simulink model "Spectrum_Analizer"  (R2022a)
settings: Solver=VariableStepAuto  StartTime=0.0  StopTime=100  RelTol=1e-3
InitFcn:
  | ts3=0.001;
  | dt=0.001;
libraries: dspsrcs4 x1, simulink x1
settings Model: Creator=TC16766  LastModifiedBy=ohadformanair
settings SolverCC: AlgebraicLoopSolver=TrustRegion
settings DebuggingCC: UnconnectedInputMsg=warning  UnconnectedOutputMsg=warning  UnconnectedLineMsg=warning  SFMachineParentedDataDiag=warning
settings RTWCC: DLArmComputeVersion=19.05

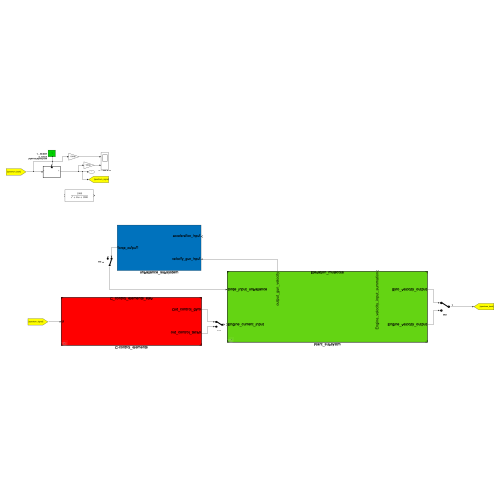
[thumbnail: Simulink's stored preview of the top-level diagram]
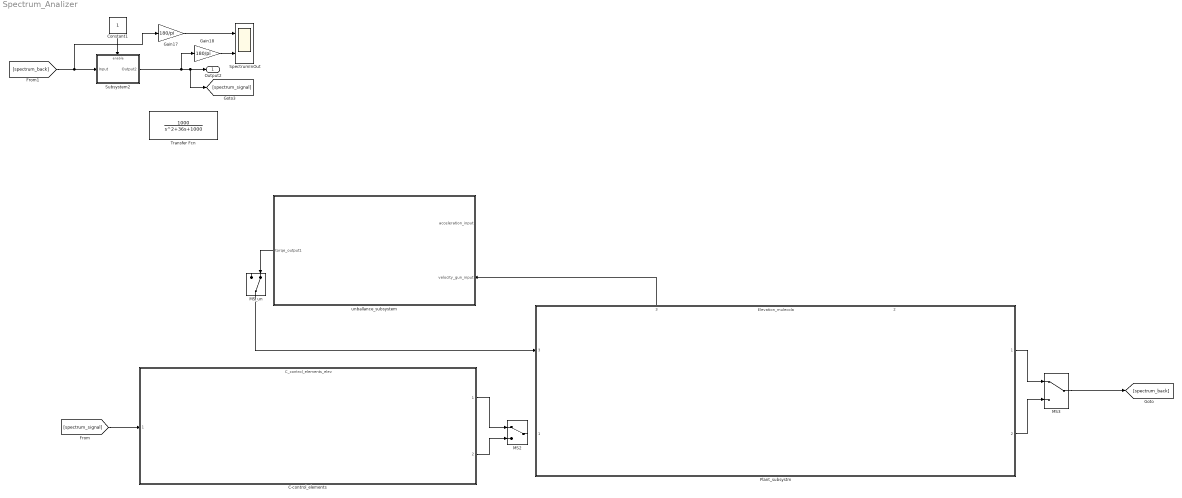
== system Spectrum_Analizer ==
  C-control_elements : ModelReference  ModelNameDialog=C_control_elements_elev  SimulationMode=Normal  ModelReferenceVersion=1.111
  Constant1 : Constant  OutDataTypeStr=boolean
      settings: AttributesFormatString=1 - START\n0 -STOP\ninternal spectrum
      settings: OpenFcn=|
      | if get_param(gcbh,'value')-48 set_param(gcbh,'value','0','backgroundcolor','red');
      | else set_param(gcbh,'value','1','backgroundcolor','green');
      | end
  Gain17 : Gain  Gain=180/pi
  Gain18 : Gain  Gain=180/pi
  MS2 : ManualSwitch
  MS3 : ManualSwitch
  MS_un : ManualSwitch  CurrentSetting=0
  Plant_subsystm : ModelReference  ModelNameDialog=Elevation_mulecola.slx  SimulationMode=Normal  ModelReferenceVersion=1.74
      settings: PortSchema="{\"entries\":[{\"content\":{\"sides\":[{\"content\":{\"connectorIds\":[\"In3\",\"In1\"]},\"type\":\"ConnectorPlacement.EquallySpacedRectSide\",\"uuid\":\"5c3be150-06c1-4b04-81d4-c89054a50b58\"},{\"content\":{\"connectorIds\":[\"Out1\",\"Out2\"],\"side\":\"RIGHT\"},\"type\":\"ConnectorPlacement.EquallySpacedRectSide\",\"uuid\":\"5dfcaa34-ef70-477d-9189-6856ebc4bbcf\"},{\"content\":{\"connectorIds\":[\"Out3\",\"In2\"],\"side\":\"TOP\"},\"type\":\"ConnectorPlacement.EquallySpacedRectSide\",\"uuid\":\"06d3d264-a507-4be0-8bff-1d5586be5fcb\"}]},\"type\":\"ConnectorPlacement.EquallySpacedConnector\",\"uuid\":\"1f4e30e1-d134-49fc-8bd6-0842cd83f06c\"}],\"packageUris\":[\"http://schema.mathworks.com/mf0/Connector/R2020b\"],\"version\":\"1.0\"}"
  SpectrumInOut : Scope  NumInputPorts=2
  Subsystem2 : Subsystem  mask{GAIN=1%2*pi/180%0.5*pi/180, InitFreq=1, TargetTime=100, FreqAtTime=100}
      mask prompts: InitFreq "INITIAL FREQUENCY"; TargetTime "Target Time"; FreqAtTime "Frequency at Time"
  Transfer Fcn : TransferFcn  Numerator=[1000]  Denominator=[1 36 1000]
  unballance_subsystem : Subsystem
      settings: PortSchema="{\"entries\":[{\"content\":{\"sides\":[{\"content\":{\"connectorIds\":[\"Out1\"]},\"type\":\"ConnectorPlacement.EquallySpacedRectSide\",\"uuid\":\"c3cd5407-f455-47fb-bed5-acab7b307edd\"},{\"content\":{\"connectorIds\":[\"In1\",\"In2\"],\"side\":\"RIGHT\"},\"type\":\"ConnectorPlacement.EquallySpacedRectSide\",\"uuid\":\"6fee87de-46ca-4c43-9525-17ad0f41a606\"},{\"content\":{\"connectorIds\":[],\"side\":\"TOP\"},\"type\":\"ConnectorPlacement.EquallySpacedRectSide\",\"uuid\":\"ba4483d7-ae58-474a-ba17-43cd832aaa5a\"},{\"content\":{\"connectorIds\":[],\"side\":\"BOTTOM\"},\"type\":\"ConnectorPlacement.EquallySpacedRectSide\",\"uuid\":\"48dc55aa-c39e-4e9a-95dc-6c3e56dde9f8\"}]},\"type\":\"ConnectorPlacement.EquallySpacedConnector\",\"uuid\":\"1afecaf5-de5a-4863-97c1-6af15bef8986\"}],\"packageUris\":[\"http://schema.mathworks.com/mf0/Connector/R2020b\"],\"version\":\"1.0\"}"
  Output2 : Outport
  wires:
  Subsystem2/1(Output2) -> [spectrum_signal], Output2/1, Gain18/1
  Gain17/1 -> SpectrumInOut/1
  Gain18/1 -> SpectrumInOut/2
  [spectrum_back] -> Gain17/1, Subsystem2/1(Input)
  Constant1/1 -> Subsystem2/Enable
  C-control_elements/2 -> MS2/2
  unballance_subsystem/1(torqe_output1) -> MS_un/2
  C-control_elements/1 -> MS2/1
  Plant_subsystm/3 -> unballance_subsystem/2(velocity_gun_input)
  MS_un/1 -> Plant_subsystm/3
  Plant_subsystm/1 -> MS3/1
  Plant_subsystm/2 -> MS3/2
  [spectrum_signal] -> C-control_elements/1
  MS3/1 -> [spectrum_back]

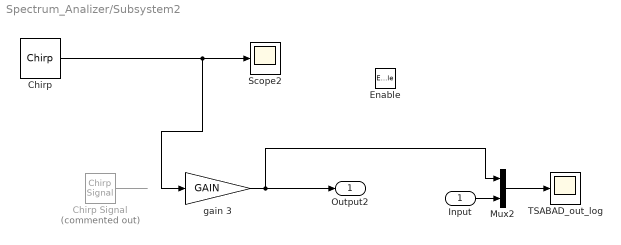
== system Spectrum_Analizer/Subsystem2 ==
  Input : Inport
  Enable : EnablePort  StatesWhenEnabling=reset
  Chirp : dspsrcs4/Chirp  sweep=Quadratic  mode=Unidirectional  f0=1  f1=FreqAtTime  t1=TargetTime  Tsweep=TargetTime  phase=0  Ts=1/100000  spf=1  datatype=Double  OutputFrames=off
  Chirp Signal : simulink/Sources/Chirp Signal  Commented=on  f1=InitFreq  T=TargetTime  f2=FreqAtTime
  Mux2 : Mux  Inputs=2
  Scope2 : Scope
  TSABAD_out_log : Scope
  gain 3 : Gain  Gain=GAIN  SaturateOnIntegerOverflow=on  SampleTime=ts3  OutDataTypeStr=Inherit: Same as input  ParamDataTypeStr=Inherit: Same as input
  Output2 : Outport
  wires:
  gain 3/1 -> Output2/1, Mux2/1
  Chirp Signal/1 -> ?
  Input/1 -> Mux2/2
  Mux2/1 -> TSABAD_out_log/1
  Chirp/1 -> gain 3/1, Scope2/1

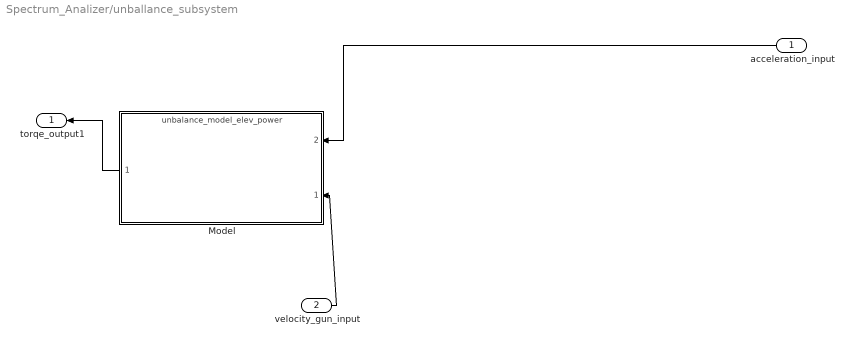
== system Spectrum_Analizer/unballance_subsystem ==
  acceleration_input : Inport
  velocity_gun_input : Inport  Port=2
  Model : ModelReference  ModelNameDialog=unbalance_model_elev_power.slx  SimulationMode=Normal  ModelReferenceVersion=1.20
      settings: PortSchema="{\"entries\":[{\"content\":{\"sides\":[{\"content\":{\"connectorIds\":[\"In2\",\"In1\"]},\"type\":\"ConnectorPlacement.EquallySpacedRectSide\",\"uuid\":\"75a92860-8d92-47f3-8dc0-8351eaabe643\"},{\"content\":{\"connectorIds\":[\"Out1\"],\"side\":\"RIGHT\"},\"type\":\"ConnectorPlacement.EquallySpacedRectSide\",\"uuid\":\"a640bfec-ecbc-4fdb-b760-0f5d774c82f6\"},{\"content\":{\"connectorIds\":[],\"side\":\"TOP\"},\"type\":\"ConnectorPlacement.EquallySpacedRectSide\",\"uuid\":\"86f4677c-440f-4e6d-a908-f26eba0e6c43\"}]},\"type\":\"ConnectorPlacement.EquallySpacedConnector\",\"uuid\":\"2beef285-55b6-492a-876b-ce1b7b923b1b\"}],\"packageUris\":[\"http://schema.mathworks.com/mf0/Connector/R2020b\"],\"version\":\"1.0\"}"
  torqe_output1 : Outport
  wires:
  velocity_gun_input/1 -> Model/1
  Model/1 -> torqe_output1/1
  acceleration_input/1 -> Model/2
